simulink model "Hornsea_anant_with_STATCOM_LIN (1)"  (R2023b)
settings: Solver=ode45  StartTime=0.0  StopTime=Tsim_lin  RelTol=1e-3
undefined symbols (not defined in the file): delta_u, sim_config, ss_sys, tstep_lin
settings Model: Creator=Josep  LastModifiedBy=Josep

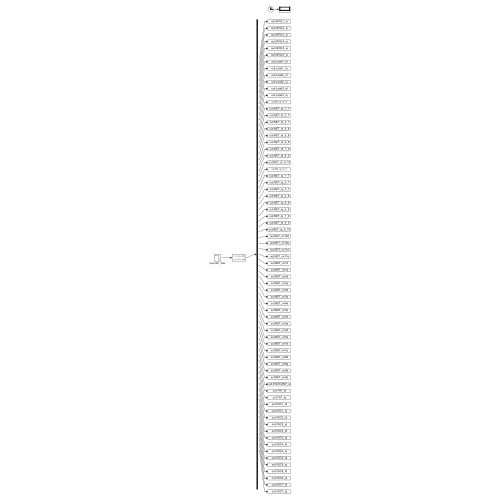
[thumbnail: Simulink's stored preview of the top-level diagram]
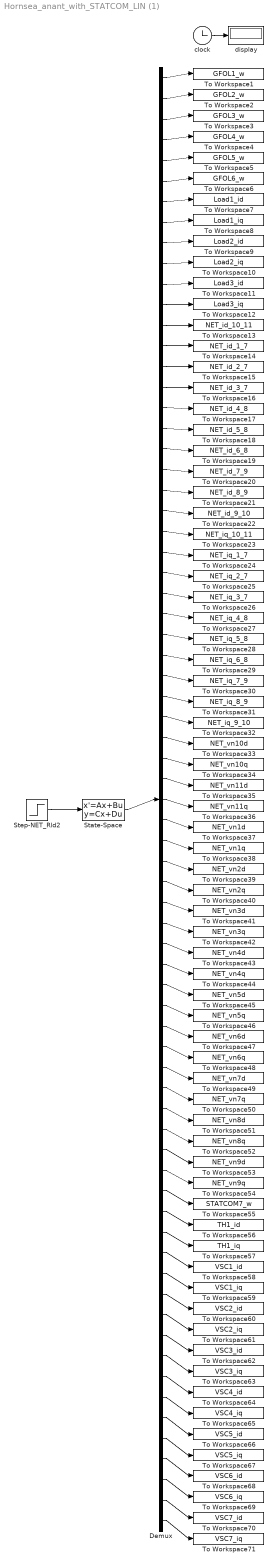
== system Hornsea_anant_with_STATCOM_LIN (1) ==
  Demux : Demux  Outputs=71
  State-Space : StateSpace  A=ss_sys.A  B=ss_sys.B  C=ss_sys.C  D=ss_sys.D  InitialCondition=0
  Step-NET_Rld2 : Step  Time=tstep_lin  After=delta_u  SampleTime=0
  To Workspace1 : ToWorkspace  VariableName=GFOL1_w  SampleTime=sim_config.Tsample
  To Workspace10 : ToWorkspace  VariableName=Load2_iq  SampleTime=sim_config.Tsample
  To Workspace11 : ToWorkspace  VariableName=Load3_id  SampleTime=sim_config.Tsample
  To Workspace12 : ToWorkspace  VariableName=Load3_iq  SampleTime=sim_config.Tsample
  To Workspace13 : ToWorkspace  VariableName=NET_id_10_11  SampleTime=sim_config.Tsample
  To Workspace14 : ToWorkspace  VariableName=NET_id_1_7  SampleTime=sim_config.Tsample
  To Workspace15 : ToWorkspace  VariableName=NET_id_2_7  SampleTime=sim_config.Tsample
  To Workspace16 : ToWorkspace  VariableName=NET_id_3_7  SampleTime=sim_config.Tsample
  To Workspace17 : ToWorkspace  VariableName=NET_id_4_8  SampleTime=sim_config.Tsample
  To Workspace18 : ToWorkspace  VariableName=NET_id_5_8  SampleTime=sim_config.Tsample
  To Workspace19 : ToWorkspace  VariableName=NET_id_6_8  SampleTime=sim_config.Tsample
  To Workspace2 : ToWorkspace  VariableName=GFOL2_w  SampleTime=sim_config.Tsample
  To Workspace20 : ToWorkspace  VariableName=NET_id_7_9  SampleTime=sim_config.Tsample
  To Workspace21 : ToWorkspace  VariableName=NET_id_8_9  SampleTime=sim_config.Tsample
  To Workspace22 : ToWorkspace  VariableName=NET_id_9_10  SampleTime=sim_config.Tsample
  To Workspace23 : ToWorkspace  VariableName=NET_iq_10_11  SampleTime=sim_config.Tsample
  To Workspace24 : ToWorkspace  VariableName=NET_iq_1_7  SampleTime=sim_config.Tsample
  To Workspace25 : ToWorkspace  VariableName=NET_iq_2_7  SampleTime=sim_config.Tsample
  To Workspace26 : ToWorkspace  VariableName=NET_iq_3_7  SampleTime=sim_config.Tsample
  To Workspace27 : ToWorkspace  VariableName=NET_iq_4_8  SampleTime=sim_config.Tsample
  To Workspace28 : ToWorkspace  VariableName=NET_iq_5_8  SampleTime=sim_config.Tsample
  To Workspace29 : ToWorkspace  VariableName=NET_iq_6_8  SampleTime=sim_config.Tsample
  To Workspace3 : ToWorkspace  VariableName=GFOL3_w  SampleTime=sim_config.Tsample
  To Workspace30 : ToWorkspace  VariableName=NET_iq_7_9  SampleTime=sim_config.Tsample
  To Workspace31 : ToWorkspace  VariableName=NET_iq_8_9  SampleTime=sim_config.Tsample
  To Workspace32 : ToWorkspace  VariableName=NET_iq_9_10  SampleTime=sim_config.Tsample
  To Workspace33 : ToWorkspace  VariableName=NET_vn10d  SampleTime=sim_config.Tsample
  To Workspace34 : ToWorkspace  VariableName=NET_vn10q  SampleTime=sim_config.Tsample
  To Workspace35 : ToWorkspace  VariableName=NET_vn11d  SampleTime=sim_config.Tsample
  To Workspace36 : ToWorkspace  VariableName=NET_vn11q  SampleTime=sim_config.Tsample
  To Workspace37 : ToWorkspace  VariableName=NET_vn1d  SampleTime=sim_config.Tsample
  To Workspace38 : ToWorkspace  VariableName=NET_vn1q  SampleTime=sim_config.Tsample
  To Workspace39 : ToWorkspace  VariableName=NET_vn2d  SampleTime=sim_config.Tsample
  To Workspace4 : ToWorkspace  VariableName=GFOL4_w  SampleTime=sim_config.Tsample
  To Workspace40 : ToWorkspace  VariableName=NET_vn2q  SampleTime=sim_config.Tsample
  To Workspace41 : ToWorkspace  VariableName=NET_vn3d  SampleTime=sim_config.Tsample
  To Workspace42 : ToWorkspace  VariableName=NET_vn3q  SampleTime=sim_config.Tsample
  To Workspace43 : ToWorkspace  VariableName=NET_vn4d  SampleTime=sim_config.Tsample
  To Workspace44 : ToWorkspace  VariableName=NET_vn4q  SampleTime=sim_config.Tsample
  To Workspace45 : ToWorkspace  VariableName=NET_vn5d  SampleTime=sim_config.Tsample
  To Workspace46 : ToWorkspace  VariableName=NET_vn5q  SampleTime=sim_config.Tsample
  To Workspace47 : ToWorkspace  VariableName=NET_vn6d  SampleTime=sim_config.Tsample
  To Workspace48 : ToWorkspace  VariableName=NET_vn6q  SampleTime=sim_config.Tsample
  To Workspace49 : ToWorkspace  VariableName=NET_vn7d  SampleTime=sim_config.Tsample
  To Workspace5 : ToWorkspace  VariableName=GFOL5_w  SampleTime=sim_config.Tsample
  To Workspace50 : ToWorkspace  VariableName=NET_vn7q  SampleTime=sim_config.Tsample
  To Workspace51 : ToWorkspace  VariableName=NET_vn8d  SampleTime=sim_config.Tsample
  To Workspace52 : ToWorkspace  VariableName=NET_vn8q  SampleTime=sim_config.Tsample
  To Workspace53 : ToWorkspace  VariableName=NET_vn9d  SampleTime=sim_config.Tsample
  To Workspace54 : ToWorkspace  VariableName=NET_vn9q  SampleTime=sim_config.Tsample
  To Workspace55 : ToWorkspace  VariableName=STATCOM7_w  SampleTime=sim_config.Tsample
  To Workspace56 : ToWorkspace  VariableName=TH1_id  SampleTime=sim_config.Tsample
  To Workspace57 : ToWorkspace  VariableName=TH1_iq  SampleTime=sim_config.Tsample
  To Workspace58 : ToWorkspace  VariableName=VSC1_id  SampleTime=sim_config.Tsample
  To Workspace59 : ToWorkspace  VariableName=VSC1_iq  SampleTime=sim_config.Tsample
  To Workspace6 : ToWorkspace  VariableName=GFOL6_w  SampleTime=sim_config.Tsample
  To Workspace60 : ToWorkspace  VariableName=VSC2_id  SampleTime=sim_config.Tsample
  To Workspace61 : ToWorkspace  VariableName=VSC2_iq  SampleTime=sim_config.Tsample
  To Workspace62 : ToWorkspace  VariableName=VSC3_id  SampleTime=sim_config.Tsample
  To Workspace63 : ToWorkspace  VariableName=VSC3_iq  SampleTime=sim_config.Tsample
  To Workspace64 : ToWorkspace  VariableName=VSC4_id  SampleTime=sim_config.Tsample
  To Workspace65 : ToWorkspace  VariableName=VSC4_iq  SampleTime=sim_config.Tsample
  To Workspace66 : ToWorkspace  VariableName=VSC5_id  SampleTime=sim_config.Tsample
  To Workspace67 : ToWorkspace  VariableName=VSC5_iq  SampleTime=sim_config.Tsample
  To Workspace68 : ToWorkspace  VariableName=VSC6_id  SampleTime=sim_config.Tsample
  To Workspace69 : ToWorkspace  VariableName=VSC6_iq  SampleTime=sim_config.Tsample
  To Workspace7 : ToWorkspace  VariableName=Load1_id  SampleTime=sim_config.Tsample
  To Workspace70 : ToWorkspace  VariableName=VSC7_id  SampleTime=sim_config.Tsample
  To Workspace71 : ToWorkspace  VariableName=VSC7_iq  SampleTime=sim_config.Tsample
  To Workspace8 : ToWorkspace  VariableName=Load1_iq  SampleTime=sim_config.Tsample
  To Workspace9 : ToWorkspace  VariableName=Load2_id  SampleTime=sim_config.Tsample
  clock : Clock
  display : Display
  wires:
  clock/1 -> display/1
  Step-NET_Rld2/1 -> State-Space/1
  State-Space/1 -> Demux/1
  Demux/1 -> To Workspace1/1
  Demux/2 -> To Workspace2/1
  Demux/3 -> To Workspace3/1
  Demux/4 -> To Workspace4/1
  Demux/5 -> To Workspace5/1
  Demux/6 -> To Workspace6/1
  Demux/7 -> To Workspace7/1
  Demux/8 -> To Workspace8/1
  Demux/9 -> To Workspace9/1
  Demux/10 -> To Workspace10/1
  Demux/11 -> To Workspace11/1
  Demux/12 -> To Workspace12/1
  Demux/13 -> To Workspace13/1
  Demux/14 -> To Workspace14/1
  Demux/15 -> To Workspace15/1
  Demux/16 -> To Workspace16/1
  Demux/17 -> To Workspace17/1
  Demux/18 -> To Workspace18/1
  Demux/19 -> To Workspace19/1
  Demux/20 -> To Workspace20/1
  Demux/21 -> To Workspace21/1
  Demux/22 -> To Workspace22/1
  Demux/23 -> To Workspace23/1
  Demux/24 -> To Workspace24/1
  Demux/25 -> To Workspace25/1
  Demux/26 -> To Workspace26/1
  Demux/27 -> To Workspace27/1
  Demux/28 -> To Workspace28/1
  Demux/29 -> To Workspace29/1
  Demux/30 -> To Workspace30/1
  Demux/31 -> To Workspace31/1
  Demux/32 -> To Workspace32/1
  Demux/33 -> To Workspace33/1
  Demux/34 -> To Workspace34/1
  Demux/35 -> To Workspace35/1
  Demux/36 -> To Workspace36/1
  Demux/37 -> To Workspace37/1
  Demux/38 -> To Workspace38/1
  Demux/39 -> To Workspace39/1
  Demux/40 -> To Workspace40/1
  Demux/41 -> To Workspace41/1
  Demux/42 -> To Workspace42/1
  Demux/43 -> To Workspace43/1
  Demux/44 -> To Workspace44/1
  Demux/45 -> To Workspace45/1
  Demux/46 -> To Workspace46/1
  Demux/47 -> To Workspace47/1
  Demux/48 -> To Workspace48/1
  Demux/49 -> To Workspace49/1
  Demux/50 -> To Workspace50/1
  Demux/51 -> To Workspace51/1
  Demux/52 -> To Workspace52/1
  Demux/53 -> To Workspace53/1
  Demux/54 -> To Workspace54/1
  Demux/55 -> To Workspace55/1
  Demux/56 -> To Workspace56/1
  Demux/57 -> To Workspace57/1
  Demux/58 -> To Workspace58/1
  Demux/59 -> To Workspace59/1
  Demux/60 -> To Workspace60/1
  Demux/61 -> To Workspace61/1
  Demux/62 -> To Workspace62/1
  Demux/63 -> To Workspace63/1
  Demux/64 -> To Workspace64/1
  Demux/65 -> To Workspace65/1
  Demux/66 -> To Workspace66/1
  Demux/67 -> To Workspace67/1
  Demux/68 -> To Workspace68/1
  Demux/69 -> To Workspace69/1
  Demux/70 -> To Workspace70/1
  Demux/71 -> To Workspace71/1
